simulink model "full_Model"  (R2023b)
settings: Solver=ode15s  StartTime=0.0  StopTime=200  RelTol=1e-3
InitFcn:
  | clear all
  | clc
  | 
  | load('EnvironmentData.mat')
  | load('userMap.mat')
  | 
  | starty = 1;
  | startx = 1;
  | endy = 20;
  | endx = 20;
  | objy = [];
  | objx = [];
  | bally = 11;
  | ballx = 11;
  | 
  | objPos=[objx,objy];
  | ballPos=[11,11,0.54];
  | boxPos=[];
  | 
  | ManipulatorSetup
  | init_quad_new_leg_raibert_strategy_v2
  | transitionMode = [-1];
values from neighbouring files (symbols this model uses):
  body = rigidBody('tool')    [InverseKinematicsV2.m]
  tar1Len = 9    [EnvironmentData.mat]
  target = [1 2.44274045536 4.0666557818 4.62742644863 6.44502800895 8.36141317519 9.41392894318 10.3865588461 10.4 10.4 11.7644392896 13.2870590067 ... (34 elements, 17x2)]    [EnvironmentData.mat]
  tarLen = 17    [EnvironmentData.mat]
undefined symbols (not defined in the file or in its folder): planner
libraries: sim3dlib x33, sharedtransform x2, visionsinks x1, visionanalysis x1, visiongeotforms x1, sim3dcameralib x1
(part 1 of 7)
settings Model: Creator=biorobotics  LastModifiedBy=olive
settings SolverCC: ZeroCrossAlgorithm=Adaptive  AlgebraicLoopSolver=TrustRegion
settings DataIOCC: ReturnWorkspaceOutputs=off
settings OptimizationCC: ReuseModelBlockBuffer=off
settings DebuggingCC: MaskedZcDiagnostic=none  IgnoredZcDiagnostic=none  UnconnectedInputMsg=warning  UnconnectedOutputMsg=warning  UnconnectedLineMsg=warning  ArithmeticOperatorsInVariantConditions=warning
settings ModelReferenceCC: EnableRefExpFcnMdlSchedulingChecks=on
settings SFSimCC: SimUseLocalCustomCode=off  CustomCodeUndefinedFunction=UseInterfaceOnly
settings RTWCC: RTWUseLocalCustomCode=off
settings DiagnosticsConfigSet: SimMechanicsRigidlyBoundBlock=none

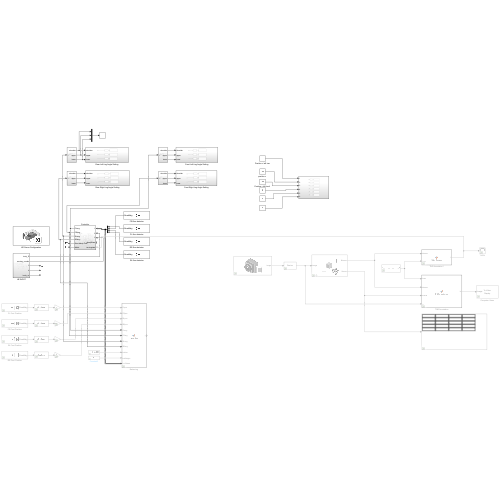
[thumbnail: Simulink's stored preview of the top-level diagram]
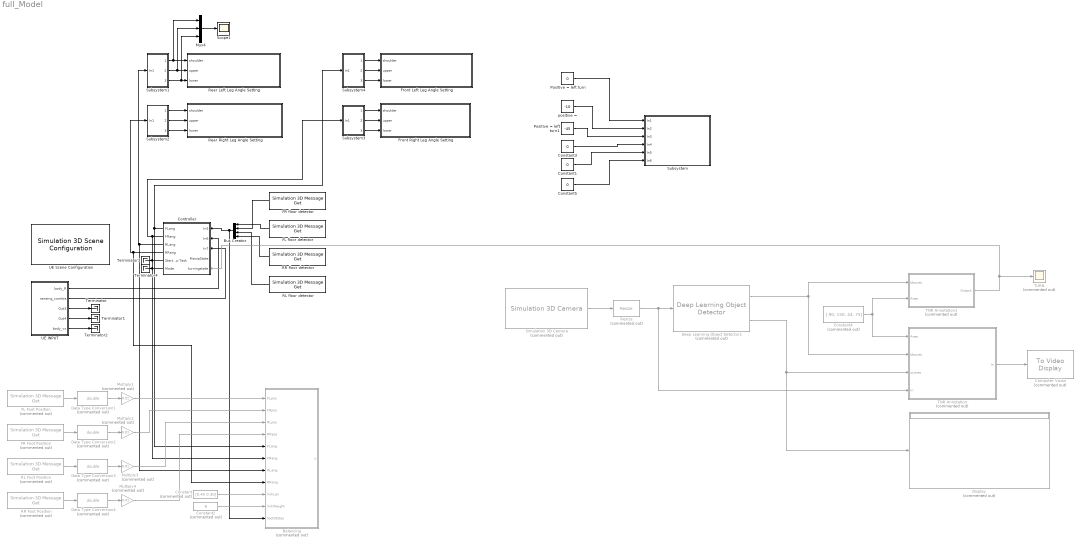
== system full_Model ==
  Balancing : MATLAB Function  Commented=on  TreatAsAtomicUnit=on
  Bus Creator : BusCreator  Inputs=4
  Computer Vision : visionsinks/To Video Display  Commented=on  windowSizeMode=Normal  openAtMdlStart=off  fullScreen=off  videoWindowX=536805376  videoWindowY=536805376  saveWindowSize=off  videoWindowWidth=1183  videoWindowHeight=779  inputColorFormat=RGB  inputType=Obsolete  imagePorts=One multidimensional signal  OutputDevice=On-screen video monitor  dataOrg=Column-major  isWindowOpen=off
  Constant : Constant  Commented=on  Value=[0.45 0.30]
  Constant1 : Constant  Value=0
  Constant2 : Constant  Commented=on  Value=8
  Constant3 : Constant  Value=0
  Constant4 : Constant  Commented=on  Value=[ 90, 150, 44, 75]  VectorParams1D=off
  Constant5 : Constant  Value=0
  Controller : Subsystem
  Data Type Conversion{1..4} (4 alike) : DataTypeConversion  Commented=on  OutDataTypeStr=double  SaturateOnIntegerOverflow=off  RndMeth=Floor
  Deep Learning Object Detector1 : visionanalysis/Deep Learning Object Detector  Commented=on  Detector=Detector from MAT-file  DetectorFunction=untitled  DetectorFilePath=C:\Year 3 Group Project\Quadruped-with-Manipulator-and-Path-Planning-10ef1b9e8f368d0d2c137c3cd991e077a3870600\Quadruped Simulink System MATLAB CODE\500DARKandSAT.mat  MaxDetections=20  Bboxes=on  Scores=on  UseROI=off  ROI=[1 1 100 100]  Threshold=0.6  NumStrongestRegions=2000  UseMinSize=off  MinSize=[1 1]  UseMaxSize=off  MaxSize=[50 50]  ForceInterpretedSim=off
  Display : Display  Commented=on
  FL Foot Position : sim3dlib/Simulation 3D Message Get  Priority=1  Commented=on  SigName=FLpositionGET  DataType=single  MsgSize=[1 3]  Ts=-1  aMode=0
      settings: LibrarySourceBlock=aerolibsim3d/Simulation 3D Message Get
  FL floor detector : sim3dlib/Simulation 3D Message Get  Priority=1  SigName=FLfloordetector  DataType=boolean  MsgSize=[1]  Ts=-1  aMode=0
      settings: LibrarySourceBlock=aerolibsim3d/Simulation 3D Message Get
  FR Foot Position : sim3dlib/Simulation 3D Message Get  Priority=1  Commented=on  SigName=FRpositionGET  DataType=single  MsgSize=[1 3]  Ts=-1  aMode=0
      settings: LibrarySourceBlock=aerolibsim3d/Simulation 3D Message Get
  FR floor detector : sim3dlib/Simulation 3D Message Get  Priority=1  SigName=FRfloordetector  DataType=boolean  MsgSize=[1]  Ts=-1  aMode=0
      settings: LibrarySourceBlock=aerolibsim3d/Simulation 3D Message Get
  Front Left Leg Angle Setting : Subsystem
  Front Right Leg Angle Setting : Subsystem
  Multiply{1..4} (4 alike) : Gain  Commented=on  Gain=0.01
  Mux4 : Mux  Inputs=3
  Positive = left turn : Constant  Value=0
  Positive = left turn1 : Constant  Value=-45
  RL Foot Position : sim3dlib/Simulation 3D Message Get  Priority=1  Commented=on  SigName=RLpositionGET  DataType=single  MsgSize=[1 3]  Ts=-1  aMode=0
      settings: LibrarySourceBlock=aerolibsim3d/Simulation 3D Message Get
  RL floor detector : sim3dlib/Simulation 3D Message Get  Priority=1  SigName=RLfloordetector  DataType=boolean  MsgSize=[1]  Ts=-1  aMode=0
      settings: LibrarySourceBlock=aerolibsim3d/Simulation 3D Message Get
  RR Foot Position : sim3dlib/Simulation 3D Message Get  Priority=1  Commented=on  SigName=RRpositionGET  DataType=single  MsgSize=[1 3]  Ts=-1  aMode=0
      settings: LibrarySourceBlock=aerolibsim3d/Simulation 3D Message Get
  RR floor detector : sim3dlib/Simulation 3D Message Get  Priority=1  SigName=RRfloordetector  DataType=boolean  MsgSize=[1]  Ts=-1  aMode=0
      settings: LibrarySourceBlock=aerolibsim3d/Simulation 3D Message Get
  Rear Left Leg Angle Setting : Subsystem
  Rear Right Leg Angle Setting : Subsystem
  Resize : visiongeotforms/Resize  Commented=on  specify=Number of output rows and columns  rfactor=[200 150]  outCols=25  outRows=25  outRowsCols=[224 224]  interp_method=Bilinear  antialias=on  useROI=off  roiFlag=off  roundingMode=Nearest  overflowMode=on  prodOutputMode=Binary point scaling  prodOutputWordLength=32  prodOutputFracLength=10
  Scope1 : Scope
  Simulation 3D Camera : sim3dcameralib/Simulation 3D Camera  Priority=1  Commented=on  sensorTag=Sim3dSensor1  sensorId=1  sensorName=Sim3dSensor1  vehTagList={'Scene Origin'}  vehTag=Scene Origin  mountLoc=Origin  offsetFlag=on  tmountOffset=[0, 0, 0.5]  extTmount=off  rmountOffset=[0, 0, 0]  extRmount=off  FocalLength=[1109, 1109]  OpticalCenter=[640, 360]  ImageSize=[720, 1280]  RadialDistortion=[0, 0]  TangentialDistortion=[0, 0]  SensorSkew=0  DepthOutportEnabled=off  SemanticOutportEnabled=off  TransformOutportEnabled=off  SampleTime=-1  mountPoint=[0 0 0.5]  mountOrientation=[0 0 0]  aMode=3  ID=1
      settings: LibrarySourceBlock=drivingsim3d/Simulation 3D Camera
  Subsystem : Subsystem
  Subsystem1 : Subsystem
  Subsystem2 : Subsystem
  Subsystem3 : Subsystem
  Subsystem4 : Subsystem
  TNR Annotation : MATLAB Function  Commented=on  TreatAsAtomicUnit=on
  TNR Annotation1 : MATLAB Function  Commented=on  TreatAsAtomicUnit=on
  TURN : Scope  Commented=on
  Terminator{,1..4} (5 alike) : Terminator
  "UE INPUT " : Subsystem
  UE Scene Configuration : sim3dlib/Simulation 3D Scene Configuration  Priority=0  ProjectFormat=Unreal Editor  SceneDesc=Empty scene  ProjectName=C:\Program Files\MATLAB\R2023b\toolbox\shared\sim3d_projects\automotive_project_windows\UE\WindowsNoEditor\VehicleSimulation.exe  ScenePath=/Game/Maps/HwStrght  UEProjPath=C:\Users\olive\Documents\Unreal Projects\Unreal Engine Project\MyProject2.uproject  EnableOpenDRIVE=off  vehTagList={'Custom';'Scene Origin'}  vehTag=Scene Origin  FreeCameraInitialTranslation=[0, 0, 0]  FreeCameraDefaultInitialTranslation=[-6, 0, 2]  FreeCameraInitialRotation=[0, 0, 0]  FreeCameraDefaultInitialRotation=[0, -15, 0]  OpVisEn=off  Ts=0.02  EnableWindow=on  EnableRemoteAccess=off  EnableWeather=off  SunAltitude=40.0  SunAzimuth=90  clouds=10  wind=1  fog=0  rain=0  EnableGeospatial=off  OriginHeight=200  OriginLatitude=40.744652  OriginLongitude=-73.988864  MapStyle=Aerial  AdditionalAssetIDs=[]  UseAdvancedSunSky=off  SolarTime=11  TimeZone=-5  Day=21  Month=9  Year=2022  UseDaylightSavingTime=on  DSTStartDay=10  DSTStartMonth=3  DSTEndDay=3  DSTEndMonth=11  DSTSwitchHour=2  sensorTag=MainCamera1  sensorId=1  sensorName=MainCamera1  mountLoc=Origin  offsetFlag=off  tmountOffset=[0, 0, 0]  rmountOffset=[0, 0, 0]  HorizontalResolution=1280  VerticalResolution=720  HorizontalFOV=60  mountPoint=[0 0 0]  mountOrientation=[0 0 0]  aMode=5  ID=1  GeoTrigger=Inactive
      settings: LibrarySourceBlock=sl3dlib/Simulation 3D/Simulation 3D Scene Configuration
  "positive = " : Constant  Value=-10
  wires:
  "UE INPUT "/1(body_R) -> Controller/2(In6)
  "UE INPUT "/4(Out4) -> Terminator1/1
  "UE INPUT "/2(sensing_combie) -> Controller/3(In7)
  "UE INPUT "/3(Out3) -> Terminator/1
  Bus Creator/1 -> Controller/1(In5), Balancing/11(footStates)
  FL floor detector/1 -> Bus Creator/1
  FR floor detector/1 -> Bus Creator/2
  RL floor detector/1 -> Bus Creator/3
  RR floor detector/1 -> Bus Creator/4
  Controller/4(RRang) -> Balancing/8(RRang), Subsystem2/1(In1)
  Controller/2(FRang) -> Subsystem3/1(In1), Balancing/6(FRang)
  Mux4/1 -> Scope1/1
  "UE INPUT "/5(body_vx) -> Terminator2/1
  Controller/5(Start Manip Task) -> Terminator3/1
  Controller/6(Mode) -> Terminator4/1
  Subsystem2/1(shoulder) -> Rear Right Leg Angle Setting/1(shoulder)
  Subsystem2/2(upper) -> Rear Right Leg Angle Setting/2(upper)
  Subsystem2/3(lower) -> Rear Right Leg Angle Setting/3(lower)
  Subsystem3/1(shoulder) -> Front Right Leg Angle Setting/1(shoulder)
  Subsystem3/2(upper) -> Front Right Leg Angle Setting/2(upper)
  Subsystem3/3(lower) -> Front Right Leg Angle Setting/3(lower)
  Subsystem1/1(shoulder) -> Mux4/1, Rear Left Leg Angle Setting/1(shoulder)
  Subsystem1/2(upper) -> Mux4/2, Rear Left Leg Angle Setting/2(upper)
  Subsystem1/3(lower) -> Mux4/3, Rear Left Leg Angle Setting/3(lower)
  Controller/3(RLang) -> Balancing/7(RLang), Subsystem1/1(In1)
  Subsystem4/1(shoulder) -> Front Left Leg Angle Setting/1(shoulder)
  Subsystem4/2(upper) -> Front Left Leg Angle Setting/2(upper)
  Subsystem4/3(lower) -> Front Left Leg Angle Setting/3(lower)
  Controller/1(FLang) -> Subsystem4/1(In1), Balancing/5(FLang)
  Simulation 3D Camera/1 -> Resize/1
  TNR Annotation1/1(Output) -> Controller/5(turningstate), TURN/1
  Constant4/1 -> TNR Annotation/1(Area), TNR Annotation1/2(Area)
  Resize/1 -> TNR Annotation/4("In "), Deep Learning Object Detector1/1
  TNR Annotation/1(In) -> Computer Vision/1
  Deep Learning Object Detector1/2 -> Display/1, TNR Annotation/3(scores)
  Deep Learning Object Detector1/1 -> TNR Annotation/2(bboxes), TNR Annotation1/1(bboxes)
  Constant3/1 -> Subsystem/4(In4)
  Constant5/1 -> Subsystem/6(In6)
  Constant1/1 -> Subsystem/5(In5)
  "positive = "/1 -> Subsystem/2(In2)
  Positive = left turn1/1 -> Subsystem/3(In3)
  Positive = left turn/1 -> Subsystem/1(In1)
  Multiply1/1 -> Balancing/1(FLpos)
  Data Type Conversion1/1 -> Multiply1/1
  FL Foot Position/1 -> Data Type Conversion1/1
  FR Foot Position/1 -> Data Type Conversion2/1
  Data Type Conversion2/1 -> Multiply2/1
  Multiply2/1 -> Balancing/2(FRpos)
  Multiply4/1 -> Balancing/4(RRpos)
  RR Foot Position/1 -> Data Type Conversion4/1
  RL Foot Position/1 -> Data Type Conversion3/1
  Data Type Conversion3/1 -> Multiply3/1
  Multiply3/1 -> Balancing/3(RLpos)
  Data Type Conversion4/1 -> Multiply4/1
  Constant/1 -> Balancing/9(linkLen)
  Constant2/1 -> Balancing/10(linkWeight)

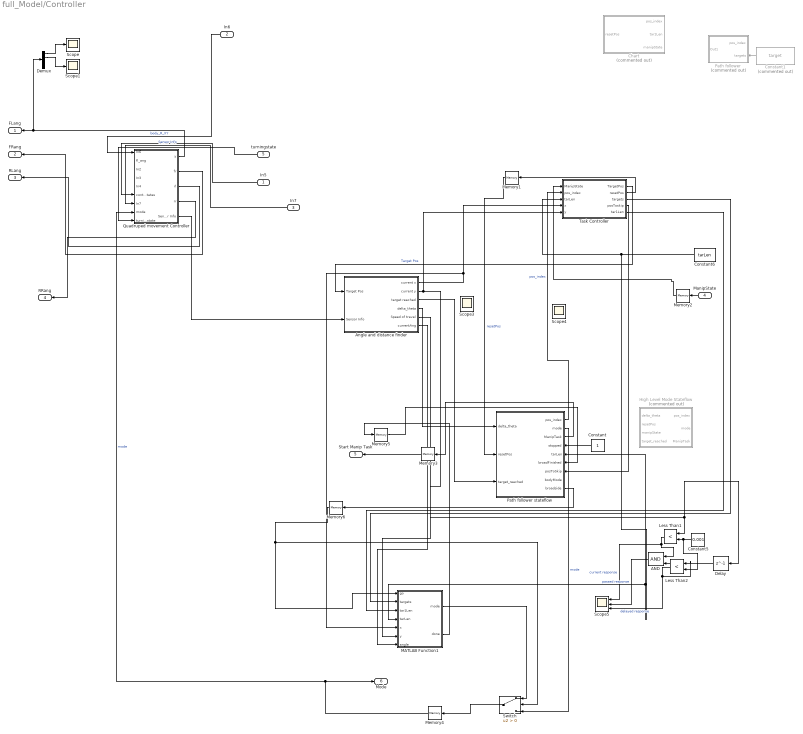
== system full_Model/Controller ==
  In5 : Inport
  In6 : Inport  Port=2
  In7 : Inport  Port=3
  ManipState : Inport  Port=4
  turningstate : Inport  Port=5
  AND : Logic  IconShape=distinctive  AllPortsSameDT=off  OutDataTypeStr=boolean
  Angle and distance finder : Subsystem
  Chart : Stateflow chart  Commented=on  TreatAsAtomicUnit=on
  Constant : Constant
  Constant1 : Constant  Commented=on  Value=target
  Constant5 : Constant  Value=0.001
  Constant6 : Constant  Value=tarLen
  Delay : Delay  DelayLength=1
  Demux : Demux
  High Level Mode Stateflow : Stateflow chart  Commented=on  TreatAsAtomicUnit=on
      settings: PortSchema="{\"entries\":[{\"content\":{\"sides\":[{\"content\":{\"connectorIds\":[\"In2\",\"In3\",\"In4\",\"In1\"]},\"type\":\"ConnectorPlacement.EquallySpacedRectSide\",\"uuid\":\"54635eaa-af22-4c07-946c-8b3764ca4079\"},{\"content\":{\"connectorIds\":[\"Out1\",\"Out2\",\"Out3\"],\"side\":\"RIGHT\"},\"type\":\"ConnectorPlacement.EquallySpacedRectSide\",\"uuid\":\"b8ca9e50-c21e-481d-aebe-d3447dd5b6ec\"},{\"content\":{\"connectorIds\":[],\"side\":\"TOP\"},\"type\":\"ConnectorPlacement.EquallySpacedRectSide\",\"uuid\":\"aa364018-0c1f-4137-8fa7-722b902e07a1\"}]},\"type\":\"ConnectorPlacement.EquallySpacedConnector\",\"uuid\":\"b87c06e7-bef4-4368-b066-66035be64295\"}],\"packageUris\":[\"http://schema.mathworks.com/mf0/Connector/R2020b\"],\"version\":\"1.0\"}"
  Less Than1 : RelationalOperator  Operator=<  OutDataTypeStr=boolean  RndMeth=Simplest  InputSameDT=off
  Less Than2 : RelationalOperator  Operator=<  OutDataTypeStr=boolean  RndMeth=Simplest  InputSameDT=off
  MATLAB Function1 : MATLAB Function  TreatAsAtomicUnit=on
  Memory{1..6} (6 alike) : Memory
  Path follower : Subsystem  Commented=on  TreatAsAtomicUnit=on
  Path follower stateflow : Stateflow chart  TreatAsAtomicUnit=on
      settings: PortSchema="{\"entries\":[{\"content\":{\"sides\":[{\"content\":{\"connectorIds\":[\"In2\",\"In3\",\"In1\"]},\"type\":\"ConnectorPlacement.EquallySpacedRectSide\",\"uuid\":\"54635eaa-af22-4c07-946c-8b3764ca4079\"},{\"content\":{\"connectorIds\":[\"Out1\",\"Out2\",\"Out3\",\"In4\",\"In5\",\"In6\",\"In7\",\"Out4\",\"Out5\"],\"side\":\"RIGHT\"},\"type\":\"ConnectorPlacement.EquallySpacedRectSide\",\"uuid\":\"b8ca9e50-c21e-481d-aebe-d3447dd5b6ec\"},{\"content\":{\"connectorIds\":[],\"side\":\"TOP\"},\"type\":\"ConnectorPlacement.EquallySpacedRectSide\",\"uuid\":\"aa364018-0c1f-4137-8fa7-722b902e07a1\"}]},\"type\":\"ConnectorPlacement.EquallySpacedConnector\",\"uuid\":\"b87c06e7-bef4-4368-b066-66035be64295\"}],\"packageUris\":[\"http://schema.mathworks.com/mf0/Connector/R2020b\"],\"version\":\"1.0\"}"
  Quadruped movement Controller : Subsystem
  Scope : Scope
  Scope1 : Scope
  Scope3 : Scope  NumInputPorts=3
  Scope4 : Scope  NumInputPorts=2
  Scope5 : Scope  NumInputPorts=3
  Switch : Switch  Criteria=u2 > Threshold  SaturateOnIntegerOverflow=off  InputSameDT=off
  Task Controller : Subsystem
  FLang : Outport  VectorParamsAs1DForOutWhenUnconnected=off
  FRang : Outport  Port=2  VectorParamsAs1DForOutWhenUnconnected=off
  RLang : Outport  Port=3  VectorParamsAs1DForOutWhenUnconnected=off
  RRang : Outport  Port=4  VectorParamsAs1DForOutWhenUnconnected=off
  Start Manip Task : Outport  Port=5  VectorParamsAs1DForOutWhenUnconnected=off
  Mode : Outport  Port=6
  wires:
  Constant6/1 -> Task Controller/3(tarLen), MATLAB Function1/4(tarLen), Path follower stateflow/5(tarLen)
  Memory1/1 -> Path follower stateflow/3(resetPos)  "resetPos"
  ManipState/1 -> Memory2/1
  Memory2/1 -> Task Controller/1(ManipState)
  Memory3/1 -> Start Manip Task/1
  Constant1/1 -> Path follower/2(targets)
  Constant5/1 -> Less Than2/2, Less Than1/2
  MATLAB Function1/2(done) -> Memory5/1
  MATLAB Function1/1(mode) -> Switch/1
  Memory4/1 -> Quadruped movement Controller/8(mode), Mode/1  "mode"
  Memory6/1 -> MATLAB Function1/1(go), Switch/2
  Switch/1 -> Memory4/1
  Memory5/1 -> Path follower stateflow/6(broadFinished)
  Path follower stateflow/1(pos_index) -> Task Controller/2(pos_index)  "pos_index"
  Path follower stateflow/3(ManipTask) -> Memory3/1
  Path follower stateflow/5(broadside) -> Memory6/1
  Path follower stateflow/2(mode) -> Switch/3  "mode"
  Task Controller/2(resetPos) -> Memory1/1
  Task Controller/3(targets) -> MATLAB Function1/2(targets)
  Task Controller/5(tar1Len) -> MATLAB Function1/3(tar1Len)
  Task Controller/4(posToskip) -> Path follower stateflow/7(posToSkip)
  Delay/1 -> Less Than2/1
  Less Than1/1 -> AND/1, Scope5/1  "current response"
  Less Than2/1 -> AND/2, Scope5/3  "delayed response"
  AND/1 -> Scope5/2  "passed response"
  Angle and distance finder/2(current y) -> Task Controller/5(y), MATLAB Function1/6(y)
  Angle and distance finder/5(Speed of travel) -> Delay/1, Less Than1/1
  Angle and distance finder/3(target reached) -> Path follower stateflow/1(target_reached)
  Angle and distance finder/1(current x) -> Task Controller/4(x), MATLAB Function1/5(x)
  Task Controller/1(TargetPos) -> Angle and distance finder/1(Target Pos)  "Target Pos"
  Angle and distance finder/4(delta_theta) -> Path follower stateflow/2(delta_theta)
  Angle and distance finder/6(currentAng) -> MATLAB Function1/7(angle)
  In6/1 -> Quadruped movement Controller/1(In6)  "body_R_XY"
  In5/1 -> Quadruped movement Controller/6(contact_states)
  In7/1 -> Quadruped movement Controller/7(In7)  "Sensor Info"
  Quadruped movement Controller/1(y) -> Demux/1, FLang/1
  Quadruped movement Controller/2(fr) -> FRang/1
  Quadruped movement Controller/3(rl) -> RLang/1
  Quadruped movement Controller/4(rr) -> RRang/1
  Quadruped movement Controller/5(Sensor Info) -> Angle and distance finder/2(Sensor Info)
  Demux/2 -> Scope1/1
  Demux/1 -> Scope/1
  Constant/1 -> Path follower stateflow/4(stopped)
  turningstate/1 -> Quadruped movement Controller/9(turningstate)

== system full_Model/Front Left Leg Angle Setting ==
  shoulder : Inport
  upper : Inport  Port=2
  lower : Inport  Port=3
  Data Type Conversion10 : DataTypeConversion  OutDataTypeStr=single  SaturateOnIntegerOverflow=off  RndMeth=Floor
  Data Type Conversion2 : DataTypeConversion  OutDataTypeStr=single  SaturateOnIntegerOverflow=off  RndMeth=Floor
  Data Type Conversion3 : DataTypeConversion  OutDataTypeStr=single  SaturateOnIntegerOverflow=off  RndMeth=Floor
  FLlower set : sim3dlib/Simulation 3D Message Set  Priority=-1  SigName=FLlower  Ts=-1  aMode=0
      settings: LibrarySourceBlock=aerolibsim3d/Simulation 3D Message Set
  FLshoulder set : sim3dlib/Simulation 3D Message Set  Priority=-1  SigName=FLshoulder  Ts=-1  aMode=0
      settings: LibrarySourceBlock=aerolibsim3d/Simulation 3D Message Set
  FLupper set : sim3dlib/Simulation 3D Message Set  Priority=-1  SigName=FLupper  Ts=-1  aMode=0
      settings: LibrarySourceBlock=aerolibsim3d/Simulation 3D Message Set
  wires:
  Data Type Conversion2/1 -> FLupper set/1
  Data Type Conversion3/1 -> FLlower set/1
  Data Type Conversion10/1 -> FLshoulder set/1
  shoulder/1 -> Data Type Conversion10/1
  upper/1 -> Data Type Conversion2/1
  lower/1 -> Data Type Conversion3/1

== system full_Model/Front Right Leg Angle Setting ==
  shoulder : Inport
  upper : Inport  Port=2
  lower : Inport  Port=3
  Data Type Conversion : DataTypeConversion  OutDataTypeStr=single  SaturateOnIntegerOverflow=off  RndMeth=Floor
  Data Type Conversion1 : DataTypeConversion  OutDataTypeStr=single  SaturateOnIntegerOverflow=off  RndMeth=Floor
  Data Type Conversion8 : DataTypeConversion  OutDataTypeStr=single  SaturateOnIntegerOverflow=off  RndMeth=Floor
  FRlower set : sim3dlib/Simulation 3D Message Set  Priority=-1  SigName=FRlower  Ts=-1  aMode=0
      settings: LibrarySourceBlock=aerolibsim3d/Simulation 3D Message Set
  FRshoulder set : sim3dlib/Simulation 3D Message Set  Priority=-1  SigName=FRshoulder  Ts=-1  aMode=0
      settings: LibrarySourceBlock=aerolibsim3d/Simulation 3D Message Set
  FRupper set : sim3dlib/Simulation 3D Message Set  Priority=-1  SigName=FRupper  Ts=-1  aMode=0
      settings: LibrarySourceBlock=aerolibsim3d/Simulation 3D Message Set
  wires:
  Data Type Conversion/1 -> FRupper set/1
  Data Type Conversion8/1 -> FRshoulder set/1
  Data Type Conversion1/1 -> FRlower set/1
  lower/1 -> Data Type Conversion1/1
  upper/1 -> Data Type Conversion/1
  shoulder/1 -> Data Type Conversion8/1

== system full_Model/Rear Left Leg Angle Setting ==
  shoulder : Inport
  upper : Inport  Port=2
  lower : Inport  Port=3
  Data Type Conversion11 : DataTypeConversion  OutDataTypeStr=single  SaturateOnIntegerOverflow=off  RndMeth=Floor
  Data Type Conversion6 : DataTypeConversion  OutDataTypeStr=single  SaturateOnIntegerOverflow=off  RndMeth=Floor
  Data Type Conversion7 : DataTypeConversion  OutDataTypeStr=single  SaturateOnIntegerOverflow=off  RndMeth=Floor
  RLlower set : sim3dlib/Simulation 3D Message Set  Priority=-1  SigName=RLlower  Ts=-1  aMode=0
      settings: LibrarySourceBlock=aerolibsim3d/Simulation 3D Message Set
  RLshoulder set : sim3dlib/Simulation 3D Message Set  Priority=-1  SigName=RLshoulder  Ts=-1  aMode=0
      settings: LibrarySourceBlock=aerolibsim3d/Simulation 3D Message Set
  RLupper set : sim3dlib/Simulation 3D Message Set  Priority=-1  SigName=RLupper  Ts=-1  aMode=0
      settings: LibrarySourceBlock=aerolibsim3d/Simulation 3D Message Set
  wires:
  Data Type Conversion6/1 -> RLupper set/1
  Data Type Conversion7/1 -> RLlower set/1
  Data Type Conversion11/1 -> RLshoulder set/1
  lower/1 -> Data Type Conversion7/1
  upper/1 -> Data Type Conversion6/1
  shoulder/1 -> Data Type Conversion11/1

== system full_Model/Rear Right Leg Angle Setting ==
  shoulder : Inport
  upper : Inport  Port=2
  lower : Inport  Port=3
  Data Type Conversion4 : DataTypeConversion  OutDataTypeStr=single  SaturateOnIntegerOverflow=off  RndMeth=Floor
  Data Type Conversion5 : DataTypeConversion  OutDataTypeStr=single  SaturateOnIntegerOverflow=off  RndMeth=Floor
  Data Type Conversion9 : DataTypeConversion  OutDataTypeStr=single  SaturateOnIntegerOverflow=off  RndMeth=Floor
  RRlower set : sim3dlib/Simulation 3D Message Set  Priority=-1  SigName=RRlower  Ts=-1  aMode=0
      settings: LibrarySourceBlock=aerolibsim3d/Simulation 3D Message Set
  RRshoulder set : sim3dlib/Simulation 3D Message Set  Priority=-1  SigName=RRshoulder  Ts=-1  aMode=0
      settings: LibrarySourceBlock=aerolibsim3d/Simulation 3D Message Set
  RRupper set : sim3dlib/Simulation 3D Message Set  Priority=-1  SigName=RRupper  Ts=-1  aMode=0
      settings: LibrarySourceBlock=aerolibsim3d/Simulation 3D Message Set
  wires:
  Data Type Conversion5/1 -> RRlower set/1
  Data Type Conversion9/1 -> RRshoulder set/1
  Data Type Conversion4/1 -> RRupper set/1
  lower/1 -> Data Type Conversion5/1
  upper/1 -> Data Type Conversion4/1
  shoulder/1 -> Data Type Conversion9/1

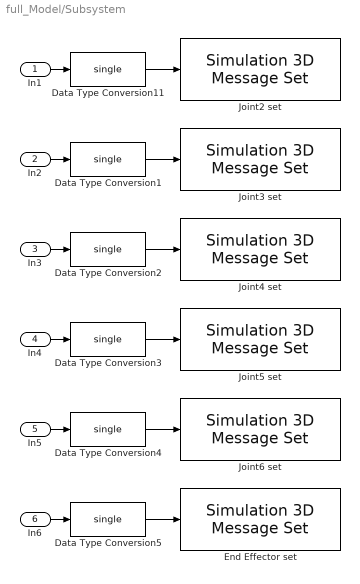
== system full_Model/Subsystem ==
  In1 : Inport
  In2 : Inport  Port=2
  In3 : Inport  Port=3
  In4 : Inport  Port=4
  In5 : Inport  Port=5
  In6 : Inport  Port=6
  Data Type Conversion{1..5,11} (6 alike) : DataTypeConversion  OutDataTypeStr=single  SaturateOnIntegerOverflow=off  RndMeth=Floor
  End Effector set : sim3dlib/Simulation 3D Message Set  Priority=-1  SigName=EndEffector  Ts=-1  aMode=0
      settings: LibrarySourceBlock=aerolibsim3d/Simulation 3D Message Set
  Joint2 set : sim3dlib/Simulation 3D Message Set  Priority=-1  SigName=ArmJoint2  Ts=-1  aMode=0
      settings: LibrarySourceBlock=aerolibsim3d/Simulation 3D Message Set
  Joint3 set : sim3dlib/Simulation 3D Message Set  Priority=-1  SigName=ArmJoint3  Ts=-1  aMode=0
      settings: LibrarySourceBlock=aerolibsim3d/Simulation 3D Message Set
  Joint4 set : sim3dlib/Simulation 3D Message Set  Priority=-1  SigName=ArmJoint4  Ts=-1  aMode=0
      settings: LibrarySourceBlock=aerolibsim3d/Simulation 3D Message Set
  Joint5 set : sim3dlib/Simulation 3D Message Set  Priority=-1  SigName=ArmJoint5  Ts=-1  aMode=0
      settings: LibrarySourceBlock=aerolibsim3d/Simulation 3D Message Set
  Joint6 set : sim3dlib/Simulation 3D Message Set  Priority=-1  SigName=ArmJoint6  Ts=-1  aMode=0
      settings: LibrarySourceBlock=aerolibsim3d/Simulation 3D Message Set
  wires:
  Data Type Conversion2/1 -> Joint4 set/1
  Data Type Conversion4/1 -> Joint6 set/1
  In5/1 -> Data Type Conversion4/1
  Data Type Conversion5/1 -> End Effector set/1
  Data Type Conversion11/1 -> Joint2 set/1
  Data Type Conversion1/1 -> Joint3 set/1
  In3/1 -> Data Type Conversion2/1
  Data Type Conversion3/1 -> Joint5 set/1
  In6/1 -> Data Type Conversion5/1
  In1/1 -> Data Type Conversion11/1
  In2/1 -> Data Type Conversion1/1
  In4/1 -> Data Type Conversion3/1

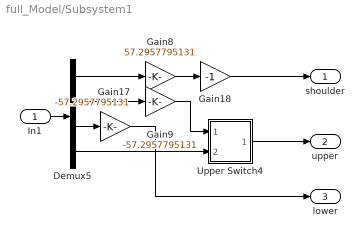
== system full_Model/Subsystem1 ==
  In1 : Inport
  Demux5 : Demux
  Gain17 : Gain  Gain=-57.2957795131
  Gain18 : Gain  Gain=-1
  Gain8 : Gain  Gain=57.2957795131
  Gain9 : Gain  Gain=-57.2957795131
  Upper Switch4 : Subsystem
  shoulder : Outport
  upper : Outport  Port=2
  lower : Outport  Port=3
  wires:
  Gain18/1 -> shoulder/1
  Demux5/1 -> Gain8/1
  Gain9/1 -> Upper Switch4/1(In1)
  Demux5/4 -> Upper Switch4/2(Input)
  Gain8/1 -> Gain18/1
  Upper Switch4/1(upper) -> upper/1
  Demux5/2 -> Gain9/1
  Demux5/3 -> Gain17/1
  In1/1 -> Demux5/1
  Gain17/1 -> lower/1

== system full_Model/Subsystem2 ==
  In1 : Inport
  Demux6 : Demux
  Gain19 : Gain  Gain=-57.2957795131
  Gain20 : Gain  Gain=-57.2957795131
  Gain21 : Gain  Gain=-57.2957795131
  Upper Switch5 : Subsystem
  shoulder : Outport
  upper : Outport  Port=2
  lower : Outport  Port=3
  wires:
  In1/1 -> Demux6/1
  Gain21/1 -> Upper Switch5/1(In1)
  Demux6/1 -> Gain19/1
  Demux6/2 -> Gain21/1
  Gain20/1 -> lower/1
  Demux6/3 -> Gain20/1
  Gain19/1 -> shoulder/1
  Upper Switch5/1(upper) -> upper/1
  Demux6/4 -> Upper Switch5/2(Input)

== system full_Model/Subsystem3 ==
  In1 : Inport
  Demux6 : Demux
  Gain19 : Gain  Gain=-57.2957795131
  Gain20 : Gain  Gain=-57.2957795131
  Gain21 : Gain  Gain=-57.2957795131
  Upper Switch5 : Subsystem
  shoulder : Outport
  upper : Outport  Port=2
  lower : Outport  Port=3
  wires:
  In1/1 -> Demux6/1
  Gain21/1 -> Upper Switch5/1(In1)
  Demux6/1 -> Gain19/1
  Demux6/2 -> Gain21/1
  Gain20/1 -> lower/1
  Demux6/3 -> Gain20/1
  Gain19/1 -> shoulder/1
  Upper Switch5/1(upper) -> upper/1
  Demux6/4 -> Upper Switch5/2(Input)

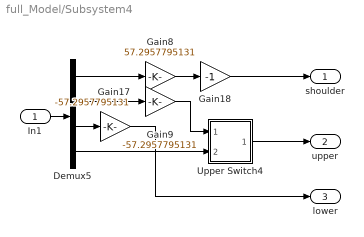
== system full_Model/Subsystem4 ==
  In1 : Inport
  Demux5 : Demux
  Gain17 : Gain  Gain=-57.2957795131
  Gain18 : Gain  Gain=-1
  Gain8 : Gain  Gain=57.2957795131
  Gain9 : Gain  Gain=-57.2957795131
  Upper Switch4 : Subsystem
  shoulder : Outport
  upper : Outport  Port=2
  lower : Outport  Port=3
  wires:
  Gain18/1 -> shoulder/1
  Demux5/1 -> Gain8/1
  Gain9/1 -> Upper Switch4/1(In1)
  Demux5/4 -> Upper Switch4/2(Input)
  Gain8/1 -> Gain18/1
  Upper Switch4/1(upper) -> upper/1
  Demux5/2 -> Gain9/1
  Demux5/3 -> Gain17/1
  In1/1 -> Demux5/1
  Gain17/1 -> lower/1

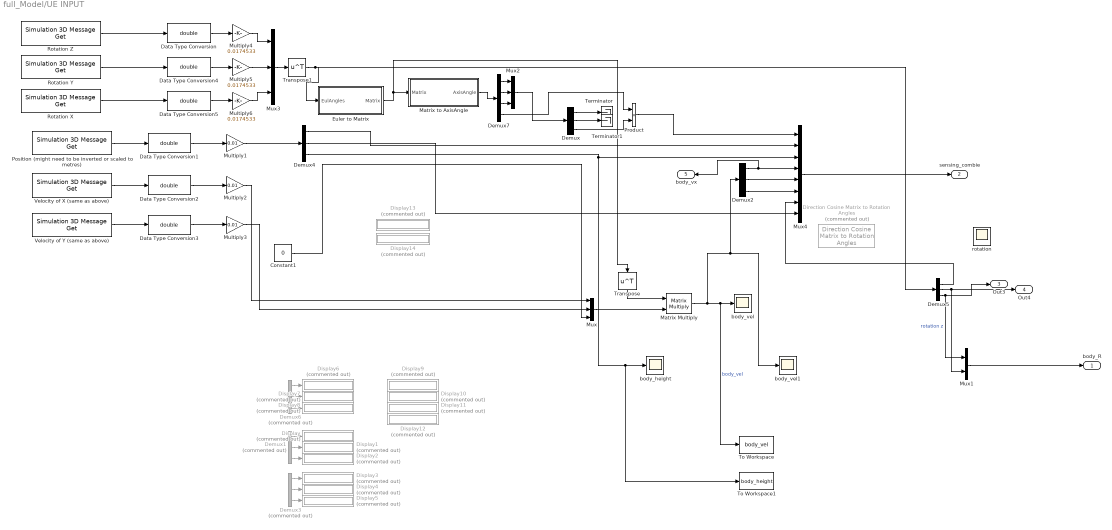
== system full_Model/UE INPUT  ==
  Constant1 : Constant  Value=0
  Data Type Conversion{,1..5} (6 alike) : DataTypeConversion  OutDataTypeStr=double  SaturateOnIntegerOverflow=off  RndMeth=Floor
  Demux{,2,4..5} (4 alike) : Demux  Outputs=3
  Demux1 : Demux  Commented=on  Outputs=3
  Demux3 : Demux  Commented=on  Outputs=3
  Demux6 : Demux  Commented=on  Outputs=3
  Demux7 : Demux
  Direction Cosine Matrix to Rotation Angles : sharedtransform/Direction Cosine Matrix to Rotation Angles  Commented=on  rotationOrder=XYZ  aMode=aMode  action=None  tolerance=eps(2)
  Display{,1..14} (15 alike) : Display  Commented=on
  Euler to Matrix : MATLAB Function  TreatAsAtomicUnit=on
  Matrix Multiply : Product  Multiplication=Matrix(*)
  Matrix to AxisAngle : MATLAB Function  TreatAsAtomicUnit=on
  Multiply1 : Gain  Gain=0.01
  Multiply2 : Gain  Gain=0.01
  Multiply3 : Gain  Gain=0.01
  Multiply4 : Gain  Gain=0.0174533
  Multiply5 : Gain  Gain=0.0174533
  Multiply6 : Gain  Gain=0.0174533
  Mux : Mux  Inputs=3
  Mux1 : Mux  Inputs=2
  Mux2 : Mux  Inputs=3
  Mux3 : Mux  Inputs=3
  Mux4 : Mux  Inputs=8
  Position (might need to be inverted or scaled to metres) : sim3dlib/Simulation 3D Message Get  Priority=1  SigName=PositionGET  DataType=single  MsgSize=[1 3]  Ts=-1  aMode=0
      settings: LibrarySourceBlock=aerolibsim3d/Simulation 3D Message Get
  Product : Product
  Rotation X : sim3dlib/Simulation 3D Message Get  Priority=1  SigName=RotationxGET  DataType=single  MsgSize=[1]  Ts=-1  aMode=0
      settings: LibrarySourceBlock=aerolibsim3d/Simulation 3D Message Get
  Rotation Y : sim3dlib/Simulation 3D Message Get  Priority=1  SigName=RotationyGET  DataType=single  MsgSize=[1]  Ts=-1  aMode=0
      settings: LibrarySourceBlock=aerolibsim3d/Simulation 3D Message Get
  Rotation Z : sim3dlib/Simulation 3D Message Get  Priority=1  SigName=RotationzGET  DataType=single  MsgSize=[1]  Ts=-1  aMode=0
      settings: LibrarySourceBlock=aerolibsim3d/Simulation 3D Message Get
  Terminator : Terminator
  Terminator1 : Terminator
  To Workspace : ToWorkspace  VariableName=body_vel  SampleTime=-1
  To Workspace1 : ToWorkspace  VariableName=body_height  SampleTime=-1
  Transpose : Math  Operator=transpose  SignedPower=on
  Transpose1 : Math  Operator=transpose
  Velocity of X (same as above) : sim3dlib/Simulation 3D Message Get  Priority=1  SigName=VectorxGET  DataType=single  MsgSize=1  Ts=-1  aMode=0
      settings: LibrarySourceBlock=aerolibsim3d/Simulation 3D Message Get
  Velocity of Y (same as above) : sim3dlib/Simulation 3D Message Get  Priority=1  SigName=VectoryGET  DataType=single  MsgSize=1  Ts=-1  aMode=0
      settings: LibrarySourceBlock=aerolibsim3d/Simulation 3D Message Get
  "body_height " : Scope
  body_vel : Scope
  body_vel1 : Scope
  "rotation " : Scope
  body_R : Outport  VectorParamsAs1DForOutWhenUnconnected=off
  sensing_combie : Outport  Port=2  VectorParamsAs1DForOutWhenUnconnected=off
  Out3 : Outport  Port=3  VectorParamsAs1DForOutWhenUnconnected=off
  Out4 : Outport  Port=4  VectorParamsAs1DForOutWhenUnconnected=off
  body_vx : Outport  Port=5
  wires:
  Mux/1 -> Matrix Multiply/2
  Mux2/1 -> Demux/1
  Mux4/1 -> sensing_combie/1
  Demux/1 -> Terminator/1
  Demux/2 -> Terminator1/1
  Demux4/1 -> Mux4/2
  Demux5/2 -> Mux1/2, Out4/1
  Demux4/3 -> To Workspace1/1, "body_height "/1, Mux4/3
  Product/1 -> Mux4/1
  Demux/3 -> Product/2
  Multiply2/1 -> Mux/1
  Demux7/4 -> Product/1
  Matrix Multiply/1 -> Demux2/1, body_vel1/1, To Workspace/1, body_vel/1  "body_vel"
  Transpose/1 -> Matrix Multiply/1
  Demux2/1 -> body_vx/1, Mux4/4
  Demux2/2 -> Mux4/5
  Demux2/3 -> Mux4/6
  Demux4/2 -> Mux4/8
  Demux7/3 -> Mux2/3
  Demux7/2 -> Mux2/2
  Demux7/1 -> Mux2/1
  Demux1/3 -> Display2/1
  Demux6/3 -> Display8/1
  Demux3/2 -> Display4/1
  Demux6/1 -> Display6/1
  Demux1/1 -> Display/1
  Demux6/2 -> Display7/1
  Matrix to AxisAngle/1(AxisAngle) -> Demux7/1
  Demux3/1 -> Display3/1
  Demux1/2 -> Display1/1
  Demux3/3 -> Display5/1
  Position (might need to be inverted or scaled to metres)/1 -> Data Type Conversion1/1
  Velocity of X (same as above)/1 -> Data Type Conversion2/1
  Mux1/1 -> body_R/1
  Euler to Matrix/1(Matrix) -> Transpose/1, Matrix to AxisAngle/1(Matrix)
  Multiply3/1 -> Mux/2
  Velocity of Y (same as above)/1 -> Data Type Conversion3/1
  Constant1/1 -> Mux/3
  Multiply4/1 -> Mux3/1
  Multiply5/1 -> Mux3/2
  Multiply6/1 -> Mux3/3
  Demux5/1 -> Mux4/7
  Demux5/3 -> Out3/1, Mux1/1  "rotation z"
  Mux3/1 -> Transpose1/1
  Transpose1/1 -> Demux5/1, Euler to Matrix/1(EulAngles)
  Data Type Conversion1/1 -> Multiply1/1
  Data Type Conversion2/1 -> Multiply2/1
  Data Type Conversion3/1 -> Multiply3/1
  Data Type Conversion/1 -> Multiply4/1
  Data Type Conversion5/1 -> Multiply6/1
  Data Type Conversion4/1 -> Multiply5/1
  Rotation X/1 -> Data Type Conversion5/1
  Rotation Y/1 -> Data Type Conversion4/1
  Rotation Z/1 -> Data Type Conversion/1
  Multiply1/1 -> Demux4/1

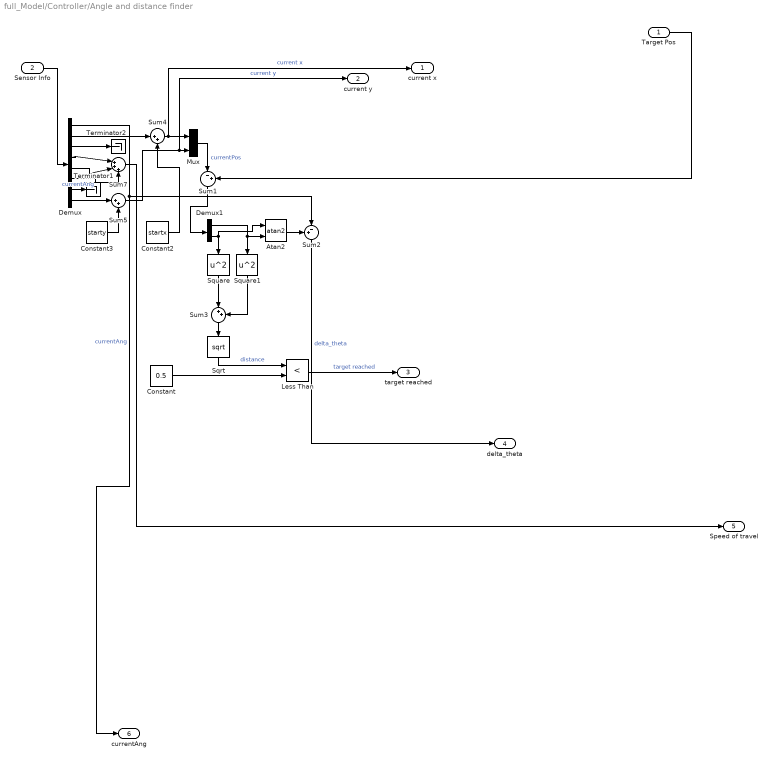
== system full_Model/Controller/Angle and distance finder ==
  Target Pos : Inport
  Sensor Info : Inport  Port=2
  Atan2 : Trigonometry  Operator=atan2
  Constant : Constant  Value=0.5
  Constant2 : Constant  Value=startx
  Constant3 : Constant  Value=starty
  Demux : Demux  Outputs=8
  Demux1 : Demux  Outputs=2
  Less Than : RelationalOperator  Operator=<  OutDataTypeStr=boolean  RndMeth=Simplest  InputSameDT=off
  Mux : Mux  Inputs=2
  Sqrt : Sqrt
  Square : Math  Operator=square
  Square1 : Math  Operator=square
  Sum1 : Sum  Inputs=|-+
  Sum2 : Sum  Inputs=+-|
  Sum3 : Sum  Inputs=|++
  Sum4 : Sum  Inputs=|++
  Sum5 : Sum  Inputs=|++
  Sum7 : Sum  Inputs=|+++
  Terminator1 : Terminator
  Terminator2 : Terminator
  current x : Outport
  current y : Outport  Port=2
  target reached : Outport  Port=3
  delta_theta : Outport  Port=4
  Speed of travel : Outport  Port=5
  currentAng : Outport  Port=6
  wires:
  Demux/5 -> Sum7/2
  Demux1/1 -> Atan2/2, Square1/1
  Square1/1 -> Sum3/2
  Demux/1 -> currentAng/1, Sum2/2  "currentAng"
  Demux1/2 -> Atan2/1, Square/1
  Constant2/1 -> Sum4/2
  Sum4/1 -> current x/1, Mux/1  "current x"
  Demux/4 -> Sum7/1
  Demux/6 -> Sum7/3
  Sqrt/1 -> Less Than/1  "distance"
  Demux/8 -> Sum5/1
  Constant3/1 -> Sum5/2
  Demux/2 -> Sum4/1
  Square/1 -> Sum3/1
  Sum5/1 -> current y/1, Mux/2  "current y"
  Demux/7 -> Terminator1/1  "currentAng"
  Sum1/1 -> Demux1/1
  Atan2/1 -> Sum2/1
  Mux/1 -> Sum1/1  "currentPos"
  Demux/3 -> Terminator2/1
  Sum3/1 -> Sqrt/1
  Constant/1 -> Less Than/2
  Less Than/1 -> target reached/1  "target reached"
  Target Pos/1 -> Sum1/2
  Sensor Info/1 -> Demux/1
  Sum7/1 -> Speed of travel/1
  Sum2/1 -> delta_theta/1  "delta_theta"

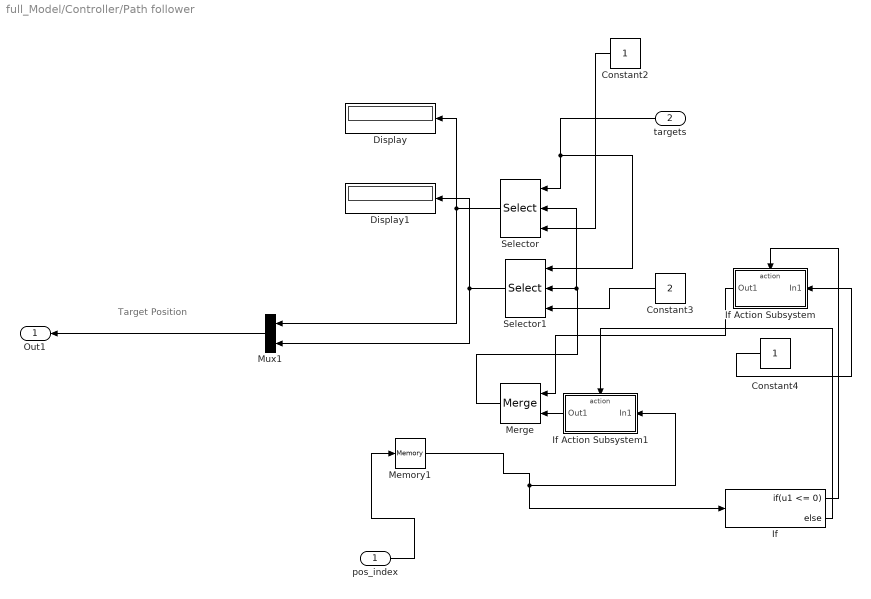
== system full_Model/Controller/Path follower ==
  note: Target Position
  pos_index : Inport
  targets : Inport  Port=2
  Constant2 : Constant
  Constant3 : Constant  Value=2
  Constant4 : Constant
  Display : Display
  Display1 : Display
  If : If  IfExpression=u1 <= 0
  If Action Subsystem : Subsystem  TreatAsAtomicUnit=on
  If Action Subsystem1 : Subsystem  TreatAsAtomicUnit=on
  Memory1 : Memory
  Merge : Merge
  Mux1 : Mux  Inputs=2
  Selector : Selector  NumberOfDimensions=2  InputPortWidth=1  IndexOptions=Index vector (port),Index vector (port)  Indices=[1 3],1  OutputSizes=1,1
  Selector1 : Selector  NumberOfDimensions=2  InputPortWidth=1  IndexOptions=Index vector (port),Index vector (port)  Indices=[1 3],1  OutputSizes=1,1
  Out1 : Outport
  wires:
  If/1 -> If Action Subsystem/Action
  Constant4/1 -> If Action Subsystem/1(In1)
  Merge/1 -> Selector/2, Selector1/2
  Memory1/1 -> If Action Subsystem1/1(In1), If/1
  Selector/1 -> Mux1/1, Display/1
  Selector1/1 -> Display1/1, Mux1/2
  targets/1 -> Selector1/1, Selector/1
  If Action Subsystem1/1(Out1) -> Merge/2
  If/2 -> If Action Subsystem1/Action
  Constant2/1 -> Selector/3
  If Action Subsystem/1(Out1) -> Merge/1
  Mux1/1 -> Out1/1
  Constant3/1 -> Selector1/3
  pos_index/1 -> Memory1/1

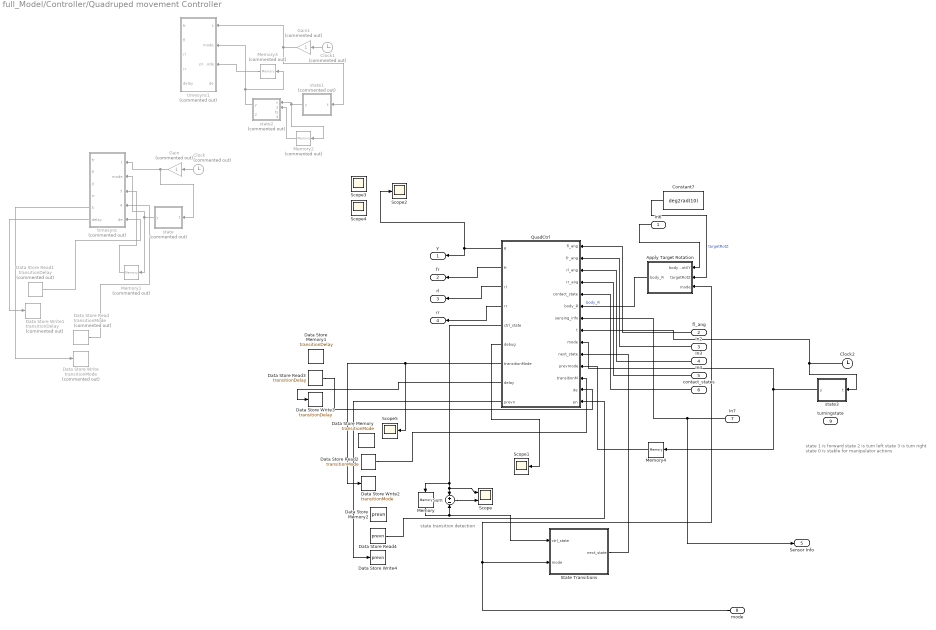
== system full_Model/Controller/Quadruped movement Controller ==
  note: state transition detection
  note: state 1 is forward
      | state 2 is turn left
      | state 3 is turn right
      |
      | state 0 is stable for manipulator actions
  In6 : Inport
  fl_ang : Inport  Port=2
  In2 : Inport  Port=3
  In3 : Inport  Port=4
  In4 : Inport  Port=5
  contact_states : Inport  Port=6
  In7 : Inport  Port=7
  mode : Inport  Port=8
  turningstate : Inport  Port=9
  Apply Target Rotation : Subsystem
  Clock : Clock  Commented=on
  Clock1 : Clock  Commented=on
  Clock2 : Clock
  Constant7 : Constant  Value=deg2rad(10)
  Data Store Memory : DataStoreMemory  DataStoreName=transitionMode  WriteAfterWriteMsg=warning  InitialValue=-1  ShowAdditionalParam=off  OutDataTypeStr=double
  Data Store Memory1 : DataStoreMemory  DataStoreName=transitionDelay  WriteAfterWriteMsg=warning  ShowAdditionalParam=off  OutDataTypeStr=double
  Data Store Memory2 : DataStoreMemory  DataStoreName=prevn  WriteAfterWriteMsg=warning  InitialValue=1  ShowAdditionalParam=off  OutDataTypeStr=double
  Data Store Read : DataStoreRead  Commented=on  DataStoreName=transitionMode  IndexOptions=Index vector (dialog)  Indices=1  OutputSizes=1
  Data Store Read1 : DataStoreRead  Commented=on  DataStoreName=transitionDelay  IndexOptions=Index vector (dialog)  Indices=1  OutputSizes=1
  Data Store Read2 : DataStoreRead  DataStoreName=transitionMode  IndexOptions=Index vector (dialog)  Indices=1  OutputSizes=1
  Data Store Read3 : DataStoreRead  DataStoreName=transitionDelay  IndexOptions=Index vector (dialog)  Indices=1  OutputSizes=1
  Data Store Read4 : DataStoreRead  DataStoreName=prevn  IndexOptions=Index vector (dialog)  Indices=1  OutputSizes=1
  Data Store Write : DataStoreWrite  Commented=on  DataStoreName=transitionMode  IndexOptions=Index vector (dialog)  Indices=1  OutputSizes=1
  Data Store Write1 : DataStoreWrite  Commented=on  DataStoreName=transitionDelay  IndexOptions=Index vector (dialog)  Indices=1  OutputSizes=1
  Data Store Write2 : DataStoreWrite  DataStoreName=transitionMode  IndexOptions=Index vector (dialog)  Indices=1  OutputSizes=1
  Data Store Write3 : DataStoreWrite  DataStoreName=transitionDelay  IndexOptions=Index vector (dialog)  Indices=1  OutputSizes=1
  Data Store Write4 : DataStoreWrite  DataStoreName=prevn  IndexOptions=Index vector (dialog)  Indices=1  OutputSizes=1
  Gain : Gain  Commented=on
  Gain1 : Gain  Commented=on
  Memory : Memory
  Memory1 : Memory  Commented=on
  Memory2 : Memory  Commented=on
  Memory3 : Memory  Commented=on
  Memory4 : Memory
  QuadCtrl : MATLAB Function  TreatAsAtomicUnit=on  SystemSampleTime=0.0025
  Scope : Scope  NumInputPorts=2
  Scope{1..5} (5 alike) : Scope
  State Transitions : Stateflow chart  TreatAsAtomicUnit=on
  Sum : Sum  Inputs=+-
  state : MATLAB Function  Commented=on  TreatAsAtomicUnit=on
  state1 : MATLAB Function  Commented=on  TreatAsAtomicUnit=on
  state2 : MATLAB Function  Commented=on  TreatAsAtomicUnit=on
  state3 : MATLAB Function  TreatAsAtomicUnit=on
  timesync : MATLAB Function  Commented=on  TreatAsAtomicUnit=on
  timesync1 : MATLAB Function  Commented=on  TreatAsAtomicUnit=on
  y : Outport  VectorParamsAs1DForOutWhenUnconnected=off
  fr : Outport  Port=2  VectorParamsAs1DForOutWhenUnconnected=off
  rl : Outport  Port=3  VectorParamsAs1DForOutWhenUnconnected=off
  rr : Outport  Port=4  VectorParamsAs1DForOutWhenUnconnected=off
  Sensor Info : Outport  Port=5
  wires:
  mode/1 -> Apply Target Rotation/3(mode), State Transitions/2(mode)
  Memory/1 -> State Transitions/1(ctrl_state), Sum/2
  Sum/1 -> Scope/2
  In2/1 -> QuadCtrl/2(fr_ang)
  State Transitions/1(next_state) -> QuadCtrl/10(next_state)
  contact_states/1 -> QuadCtrl/5(contact_state)
  In3/1 -> QuadCtrl/3(rl_ang)
  In6/1 -> Apply Target Rotation/1(body_RotXY)
  QuadCtrl/6(debug) -> Scope1/1
  Constant7/1 -> Apply Target Rotation/2(targetRotZ)  "targetRotZ"
  Apply Target Rotation/1(body_R) -> QuadCtrl/6(body_R)  "body_R"
  In7/1 -> Sensor Info/1, QuadCtrl/7(sensing_info)
  QuadCtrl/5(ctrl_state) -> Scope/1, Sum/1, Memory/1
  In4/1 -> QuadCtrl/4(rr_ang)
  Clock/1 -> Gain/1
  Gain/1 -> timesync/1(t), state/1(t)
  state/1(y) -> timesync/2(mode), Memory1/1
  Memory1/1 -> timesync/3(prevmode)
  Clock1/1 -> Gain1/1
  Gain1/1 -> state1/1(t), timesync1/1(t)
  state1/1(y) -> Memory2/1, state2/1(x)
  state2/1(y) -> timesync1/2(mode), Memory3/1
  Memory2/1 -> state2/2(prev_x)
  Memory3/1 -> timesync1/3(prevmode)
  Data Store Read1/1 -> timesync/5(de)
  timesync/6(delay) -> Data Store Write1/1
  Data Store Read/1 -> timesync/4(transitionM)
  timesync/5(transitionMode) -> Data Store Write/1
  QuadCtrl/2(fr) -> fr/1
  QuadCtrl/1(fl) -> y/1, Scope2/1
  QuadCtrl/3(rl) -> rl/1
  QuadCtrl/4(rr) -> rr/1
  QuadCtrl/8(delay) -> Data Store Write3/1
  QuadCtrl/7(transitionMode) -> Scope5/1, Data Store Write2/1
  Data Store Read2/1 -> QuadCtrl/12(transitionM)
  Data Store Read3/1 -> QuadCtrl/13(de)
  Clock2/1 -> QuadCtrl/8(t), state3/1(t)
  Memory4/1 -> QuadCtrl/11(prevmode)
  fl_ang/1 -> QuadCtrl/1(fl_ang)
  Data Store Read4/1 -> QuadCtrl/14(pn)
  QuadCtrl/9(prevn) -> Data Store Write4/1
  state3/1(y) -> Memory4/1, QuadCtrl/9(mode)

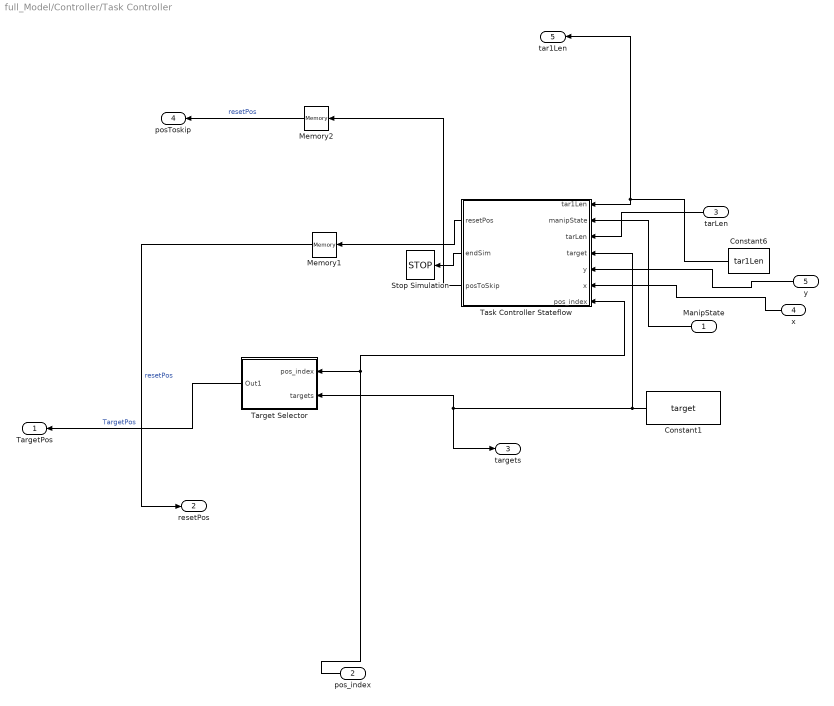
== system full_Model/Controller/Task Controller ==
  ManipState : Inport
  pos_index : Inport  Port=2
  tarLen : Inport  Port=3
  x : Inport  Port=4
  y : Inport  Port=5
  Constant1 : Constant  Value=target
  Constant6 : Constant  Value=tar1Len
  Memory1 : Memory
  Memory2 : Memory
  Stop Simulation : Stop
  Target Selector : Subsystem  TreatAsAtomicUnit=on
  Task Controller Stateflow : Stateflow chart  TreatAsAtomicUnit=on
  TargetPos : Outport
  resetPos : Outport  Port=2
  targets : Outport  Port=3
  posToskip : Outport  Port=4
  tar1Len : Outport  Port=5
  wires:
  tarLen/1 -> Task Controller Stateflow/3(tarLen)
  pos_index/1 -> Task Controller Stateflow/7(pos_index), Target Selector/1(pos_index)
  Task Controller Stateflow/2(endSim) -> Stop Simulation/1
  ManipState/1 -> Task Controller Stateflow/2(manipState)
  Task Controller Stateflow/1(resetPos) -> Memory1/1
  Memory1/1 -> resetPos/1  "resetPos"
  Constant1/1 -> targets/1, Target Selector/2(targets), Task Controller Stateflow/4(target)
  Constant6/1 -> tar1Len/1, Task Controller Stateflow/1(tar1Len)
  Target Selector/1(Out1) -> TargetPos/1  "TargetPos"
  Task Controller Stateflow/3(posToSkip) -> Memory2/1
  Memory2/1 -> posToskip/1  "resetPos"
  y/1 -> Task Controller Stateflow/5(y)
  x/1 -> Task Controller Stateflow/6(x)

== system full_Model/Subsystem1/Upper Switch4 ==
  In1 : Inport
  Input : Inport  Port=2
  Memory : Memory  InitialCondition=-33  InheritSampleTime=on
  Switch : Switch  Criteria=u2 > Threshold  SaturateOnIntegerOverflow=off  InputSameDT=off
  upper : Outport
  wires:
  In1/1 -> Switch/1
  Memory/1 -> Switch/3
  Input/1 -> Switch/2
  Switch/1 -> Memory/1, upper/1

== system full_Model/Subsystem2/Upper Switch5 ==
  In1 : Inport
  Input : Inport  Port=2
  Memory : Memory  InitialCondition=-33  InheritSampleTime=on
  Switch : Switch  Criteria=u2 > Threshold  SaturateOnIntegerOverflow=off  InputSameDT=off
  upper : Outport
  wires:
  Switch/1 -> Memory/1, upper/1
  Input/1 -> Switch/2
  In1/1 -> Switch/1
  Memory/1 -> Switch/3

== system full_Model/Subsystem3/Upper Switch5 ==
  In1 : Inport
  Input : Inport  Port=2
  Memory : Memory  InitialCondition=-33  InheritSampleTime=on
  Switch : Switch  Criteria=u2 > Threshold  SaturateOnIntegerOverflow=off  InputSameDT=off
  upper : Outport
  wires:
  Switch/1 -> Memory/1, upper/1
  Input/1 -> Switch/2
  In1/1 -> Switch/1
  Memory/1 -> Switch/3

== system full_Model/Subsystem4/Upper Switch4 ==
  In1 : Inport
  Input : Inport  Port=2
  Memory : Memory  InitialCondition=-33  InheritSampleTime=on
  Switch : Switch  Criteria=u2 > Threshold  SaturateOnIntegerOverflow=off  InputSameDT=off
  upper : Outport
  wires:
  In1/1 -> Switch/1
  Memory/1 -> Switch/3
  Input/1 -> Switch/2
  Switch/1 -> Memory/1, upper/1

== system full_Model/Controller/Path follower/If Action Subsystem ==
  In1 : Inport
  Action Port : ActionPort  ActionPortLabel=if(u1 <= 0)
  Out1 : Outport
  wires:
  In1/1 -> Out1/1

== system full_Model/Controller/Path follower/If Action Subsystem1 ==
  In1 : Inport
  Action Port : ActionPort  ActionPortLabel=else
  Out1 : Outport
  wires:
  In1/1 -> Out1/1

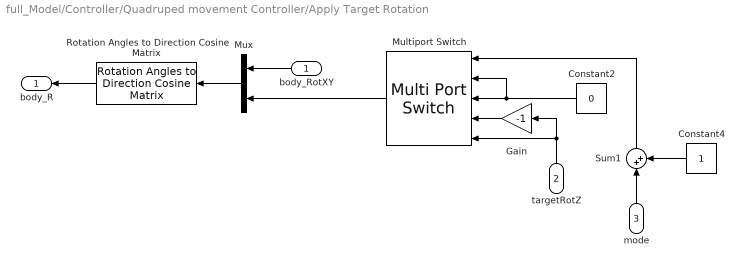
== system full_Model/Controller/Quadruped movement Controller/Apply Target Rotation ==
  body_RotXY : Inport
  targetRotZ : Inport  Port=2
  mode : Inport  Port=3
  Constant2 : Constant  Value=0
  Constant4 : Constant
  Gain : Gain  Gain=-1
  Multiport Switch : MultiPortSwitch  Inputs=4  SaturateOnIntegerOverflow=off  InputSameDT=off
  Mux : Mux  Inputs=2
  Rotation Angles to Direction Cosine Matrix : sharedtransform/Rotation Angles to Direction Cosine Matrix  rotationOrder=XYZ  aMode=aMode
  Sum1 : Sum  Inputs=|++
  body_R : Outport
  wires:
  Mux/1 -> Rotation Angles to Direction Cosine Matrix/1
  targetRotZ/1 -> Multiport Switch/5, Gain/1
  Multiport Switch/1 -> Mux/2
  Constant2/1 -> Multiport Switch/2, Multiport Switch/3
  Sum1/1 -> Multiport Switch/1
  Constant4/1 -> Sum1/2
  Gain/1 -> Multiport Switch/4
  body_RotXY/1 -> Mux/1
  Rotation Angles to Direction Cosine Matrix/1 -> body_R/1
  mode/1 -> Sum1/1

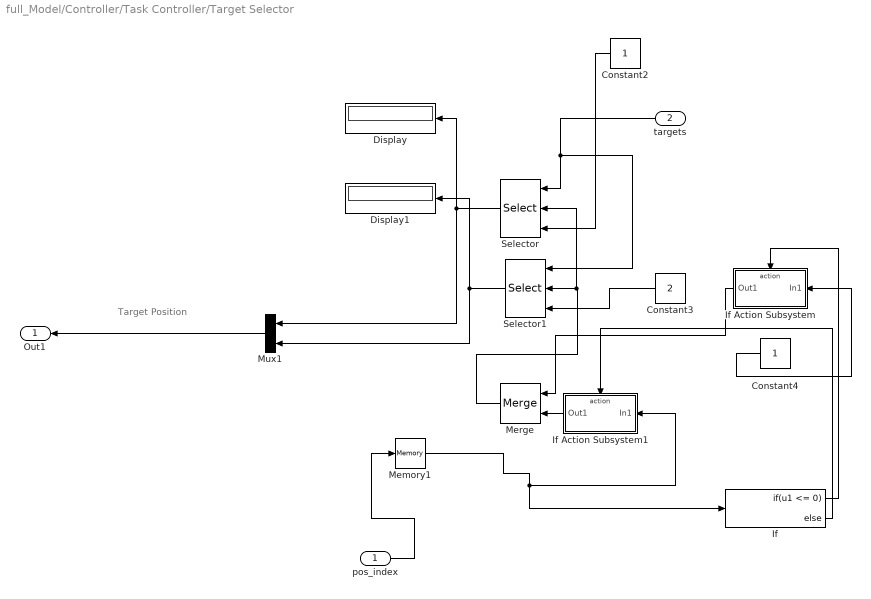
== system full_Model/Controller/Task Controller/Target Selector ==
  note: Target Position
  pos_index : Inport
  targets : Inport  Port=2
  Constant2 : Constant
  Constant3 : Constant  Value=2
  Constant4 : Constant
  Display : Display
  Display1 : Display
  If : If  IfExpression=u1 <= 0
  If Action Subsystem : Subsystem  TreatAsAtomicUnit=on
  If Action Subsystem1 : Subsystem  TreatAsAtomicUnit=on
  Memory1 : Memory
  Merge : Merge
  Mux1 : Mux  Inputs=2
  Selector : Selector  NumberOfDimensions=2  InputPortWidth=1  IndexOptions=Index vector (port),Index vector (port)  Indices=[1 3],1  OutputSizes=1,1
  Selector1 : Selector  NumberOfDimensions=2  InputPortWidth=1  IndexOptions=Index vector (port),Index vector (port)  Indices=[1 3],1  OutputSizes=1,1
  Out1 : Outport
  wires:
  If/1 -> If Action Subsystem/Action
  Constant4/1 -> If Action Subsystem/1(In1)
  Merge/1 -> Selector/2, Selector1/2
  Memory1/1 -> If Action Subsystem1/1(In1), If/1
  Selector/1 -> Mux1/1, Display/1
  Selector1/1 -> Display1/1, Mux1/2
  targets/1 -> Selector1/1, Selector/1
  If Action Subsystem1/1(Out1) -> Merge/2
  If/2 -> If Action Subsystem1/Action
  Constant2/1 -> Selector/3
  If Action Subsystem/1(Out1) -> Merge/1
  Mux1/1 -> Out1/1
  Constant3/1 -> Selector1/3
  pos_index/1 -> Memory1/1

== system full_Model/Controller/Task Controller/Target Selector/If Action Subsystem ==
  In1 : Inport
  Action Port : ActionPort  ActionPortLabel=if(u1 <= 0)
  Out1 : Outport
  wires:
  In1/1 -> Out1/1

== system full_Model/Controller/Task Controller/Target Selector/If Action Subsystem1 ==
  In1 : Inport
  Action Port : ActionPort  ActionPortLabel=else
  Out1 : Outport
  wires:
  In1/1 -> Out1/1

== stateflow chart full_Model/Controller/Quadruped movement Controller/State Transitions ==
  state Initilisation
    next_state = 1;
  state Walking_Phase_fr_rl
    next_state = 2;
  state Stationary
    next_state = 4;
  state Walking_Phase_fl_rr
    next_state = 3;
  (default) -> Initilisation
  Initilisation -> Stationary : [ctrl_state==next_state]
  Stationary -> Walking_Phase_fr_rl : [mode >= 1 && ctrl_state == next_state]
  Walking_Phase_fl_rr -> Walking_Phase_fr_rl [order 2] : [ctrl_state == next_state]
  Walking_Phase_fr_rl -> (junction 49) [order 1] : [mode == 0]
  Walking_Phase_fr_rl -> Walking_Phase_fl_rr [order 2] : [ctrl_state == next_state]
  (junction 49) -> Stationary
  Walking_Phase_fl_rr -> (junction 49) [order 1] : [mode == 0]
  data: ctrl_state input =0; mode input =0; next_state output
